simulink model "batteryGridPV_v17"  (R2014a)
settings: Solver=ode23tb  StartTime=0.0  StopTime=86400  MaxStep=0.2  RelTol=1e-5
PreLoadFcn:
  | % -- Recommended Settings --
  | %
  | %  Simulink:
  | %      Solver: Ode23tb
  | %      Relative tolerance = 1e-4
  | %      Max step size = 0.2
  | %
  | %  Powergui:
  |          Ts = 0; % (continuous electrical model)
  | %
  | %
  | % ----------------------------------
InitFcn:
  | Ncell = 80;
  | PVCellIsc = 7;
  | PVCellVoc = 0.64;
  | PVCellRs = 0.001;
  | tau = 1e-4;
  | 
  | initializeBattery();
StopFcn:
  | %plotSimResults();
values from neighbouring files (symbols this model uses):
  ambientTemp = 20    [initialConditions.m]    (also in initializeBattery.m)
  currentSat = 0.5    [controlParams.m]    (also in initializeBattery.m)
  desiredBusVoltage = 30    [controlParams.m]    (also in initializeBattery.m = 24.45)
  finalVoltage = 30    [controlParams.m]    (also in initializeBattery.m = 26)
  maxChargeRate = 5    [controlParams.m]    (also in initializeBattery.m)
  maxDischargeRate = -5    [controlParams.m]    (also in initializeBattery.m)
  T_init = ambientTemp + 273.15    (= 293.15)    [initialConditions.m]    (also in initializeBattery.m)
undefined symbols (not defined in the file or in its folder): Ion, Lithium
undefined symbols (not defined in the file): C1_LUT, C2_LUT, Capacity_LUT, cell_Cp_heat, cell_mass, Em_LUT, Qe_init, R0_LUT, R1_LUT, R2_LUT, SOC_LUT, Temperature_LUT
libraries: powerlib x42, fl_lib x18, nesl_utility x6, LiBatteryElements_lib x6, simulink x3, simulink_extras x3, electricdrivelib x1
(part 2 of 2)

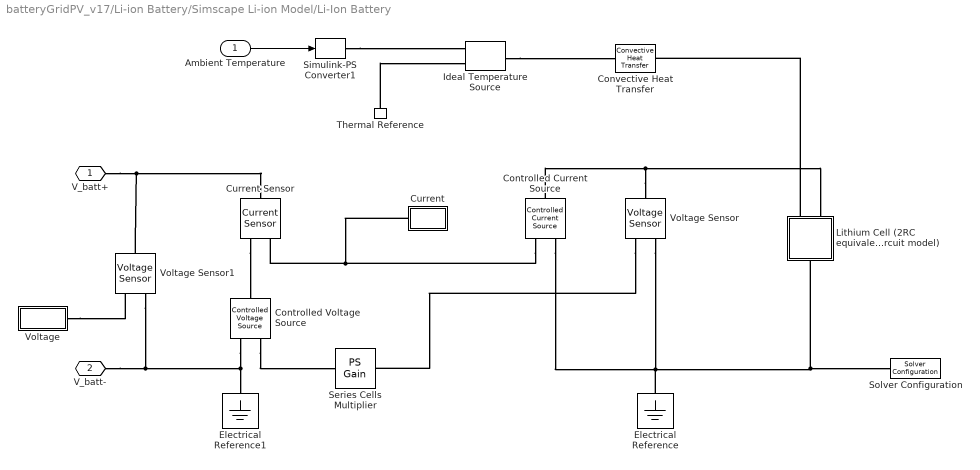
== system batteryGridPV_v17/Li-ion Battery/Simscape Li-ion Model/Li-Ion Battery ==
  Ambient Temperature : Inport
  Controlled Current Source : fl_lib/Electrical/Electrical Sources/Controlled Current Source
  Controlled Voltage Source : fl_lib/Electrical/Electrical Sources/Controlled Voltage Source
  Convective Heat Transfer : fl_lib/Thermal/Thermal Elements/Convective Heat Transfer  area=cell_area m^2  heat_tr_coeff=h_conv W/(m^2 * K)  Q_specify=off  Q_priority=High  Q=0 J/s  T_specify=off  T_priority=High  T=0 K
  Current : Subsystem
  Current Sensor : fl_lib/Electrical/Electrical Sensors/Current Sensor
  Electrical Reference : fl_lib/Electrical/Electrical Elements/Electrical Reference
  Electrical Reference1 : fl_lib/Electrical/Electrical Elements/Electrical Reference
  Ideal Temperature Source : fl_lib/Thermal/Thermal Sources/Ideal Temperature Source
  Lithium Cell (2RC equivalent circuit model) : Subsystem  mask(Lithium battery (two RC-branch equivalent circuit)){Qe_init=Qe_init, T_init=T_init, Capacity_LUT=Capacity_LUT, Em_LUT=Em_LUT, R0_LUT=R0_LUT, R1_LUT=R1_LUT, C1_LUT=C1_LUT, R2_LUT=R2_LUT, C2_LUT=C2_LUT, cell_mass=cell_mass, cell_Cp_heat=cell_Cp_heat, SOC_LUT=SOC_LUT, Temperature_LUT=Temperature_LUT}
      mask prompts: Qe_init "Initial charge deficit (A*hr)"; T_init "Initial cell temperature (K)"; Capacity_LUT "Capacity (A*hr, 1xN table)"; Em_LUT "Em open-circuit voltage (volts, MxN table)"; R0_LUT "R0 terminal resistance (ohms, MxN table)"; R1_LUT "R1 resistance (ohms, MxN table)"; C1_LUT "C1 capacitance (farads, MxN table)"; R2_LUT "R2 resistance (ohms, MxN table)"; C2_LUT "C2 capacitance (farads, MxN table)"; cell_mass "Cell mass (kg)"; cell_Cp_heat "Cell specific heat (J/kg/K)"; SOC_LUT "SOC table breakpoints (Mx1 array)"; Temperature_LUT "Temperature table breakpoints(K, 1xN array)"
      mask Display:
      | image(imread('battery.jpg'))
      | color('red')
      | port_label('LConn',1,'H')
      | port_label('LConn',2,'+')
      | port_label('RConn',1,'-')
  Series Cells Multiplier : fl_lib/Physical Signals/Functions/PS Gain  gain=7
  Simulink-PS Converter1 : nesl_utility/Simulink-PS Converter  PhysicalDomain=network_engine_domain  SubClassName=ps_input  LeftPortType=input  RightPortType=output  PseudoPeriodic=off  Frequencies=[]  NoiseDistribution=none  NoiseParameters=[]  Unit=C  AffineConversion=on  InputFiltering=off  SimscapeFilterOrder=1  InputFilterTimeConstant=.001  UdotUserProvided=1
  Solver Configuration : nesl_utility/Solver Configuration  PhysicalDomain=network_engine_domain  SubClassName=solver  LeftPortType=input  RightPortType=generic  Accelerate=off  Tones=[]  Harmonics=[]  SimulateNoise=off  Profile=off  UseLocalSampling=off  EnableSwitchedLinearOptims=on  FrequencyDomain=off  UseCCode=off  RelTol=0.001  AbsTol=1e-06  MinStep=1e-09  ToWorkspace=off  DoDC=on  ResidualTolerance=1e-9  UseLocalSolver=off  LocalSolverChoice=NE_BACKWARD_EULER_ADVANCER  LocalSolverSampleTime=1  DoFixedCost=off  MaxNonlinIter=3  MaxModeIter=2  LinearAlgebra=Sparse  DelaysMemoryBudget=1024  AutomaticFiltering=on  FilteringTimeConstant=0.001
  Thermal Reference : fl_lib/Thermal/Thermal Elements/Thermal Reference
  Voltage : Subsystem
  Voltage Sensor : fl_lib/Electrical/Electrical Sensors/Voltage Sensor
  Voltage Sensor1 : fl_lib/Electrical/Electrical Sensors/Voltage Sensor
  V_batt+ : PMIOPort  Port=1  Side=Left
  V_batt- : PMIOPort  Port=2  Side=Left
  wires:
  Ambient Temperature/1 -> Simulink-PS Converter1/1
  connections:
  V_batt+/RConn1 -- Voltage Sensor1/LConn1 -- Current Sensor/LConn1
  Controlled Voltage Source/RConn2 -- Voltage Sensor1/RConn2 -- V_batt-/RConn1 -- Electrical Reference1/LConn1
  Lithium Cell (2RC equivalent circuit model)/LConn1 -- Convective Heat Transfer/RConn1
  Thermal Reference/LConn1 -- Ideal Temperature Source/RConn2
  Simulink-PS Converter1/RConn1 -- Ideal Temperature Source/RConn1
  Ideal Temperature Source/LConn1 -- Convective Heat Transfer/LConn1
  Electrical Reference/LConn1 -- Lithium Cell (2RC equivalent circuit model)/RConn1 -- Solver Configuration/RConn1 -- Controlled Current Source/RConn2 -- Voltage Sensor/RConn2
  Controlled Current Source/RConn1 -- Current Sensor/RConn1 -- Current/RConn1
  Controlled Voltage Source/RConn1 -- Series Cells Multiplier/RConn1
  Voltage Sensor/LConn1 -- Lithium Cell (2RC equivalent circuit model)/LConn2 -- Controlled Current Source/LConn1
  Current Sensor/RConn2 -- Controlled Voltage Source/LConn1
  Voltage Sensor/RConn1 -- Series Cells Multiplier/LConn1
  Voltage/RConn1 -- Voltage Sensor1/RConn1

== system batteryGridPV_v17/PV//Battery Power Converters/Buck Converter/scaling ==
  note: Shifting from ]0 to 1[ to a ]-1 to 1[ scale
  D : Inport
  Bias : Bias  Bias=-0.5
  Gain : Gain  Gain=2
  Saturation : Saturate  UpperLimit=1  LowerLimit=-1
  m : Outport
  wires:
  Bias/1 -> Gain/1
  D/1 -> Bias/1
  Gain/1 -> Saturation/1
  Saturation/1 -> m/1

== system batteryGridPV_v17/Battery//PV Management and Control/Battery Charge//Discharge Controllers/Battery Charge Controller/scaling ==
  note: Shifting from ]0 to 1[ to a ]-1 to 1[ scale
  D : Inport
  Bias : Bias  Bias=-0.5
  Gain : Gain  Gain=2
  Saturation : Saturate  UpperLimit=1  LowerLimit=-1
  m : Outport
  wires:
  Saturation/1 -> m/1
  Gain/1 -> Saturation/1
  D/1 -> Bias/1
  Bias/1 -> Gain/1

== system batteryGridPV_v17/Battery//PV Management and Control/Battery Charge//Discharge Controllers/Battery Discharge Controller/scaling ==
  note: Shifting from ]0 to 1[ to a ]-1 to 1[ scale
  D : Inport
  Bias : Bias  Bias=-0.5
  Gain : Gain  Gain=-2
  Saturation : Saturate  UpperLimit=1  LowerLimit=-1
  m : Outport
  wires:
  Saturation/1 -> m/1
  Gain/1 -> Saturation/1
  D/1 -> Bias/1
  Bias/1 -> Gain/1

== system batteryGridPV_v17/Li-ion Battery/Simscape Li-ion Model/Li-Ion Battery/Current ==
  PS-Simulink Converter1 : nesl_utility/PS-Simulink Converter  PhysicalDomain=network_engine_domain  SubClassName=ps_output  LeftPortType=input  RightPortType=output  PseudoPeriodic=off  Frequencies=[]  Unit=A  AffineConversion=off
  PS : PMIOPort  Port=1  Side=Right
  tag scope: I_load=global
  wires:
  PS-Simulink Converter1/1 -> [I_load]
  connections:
  PS-Simulink Converter1/LConn1 -- PS/RConn1

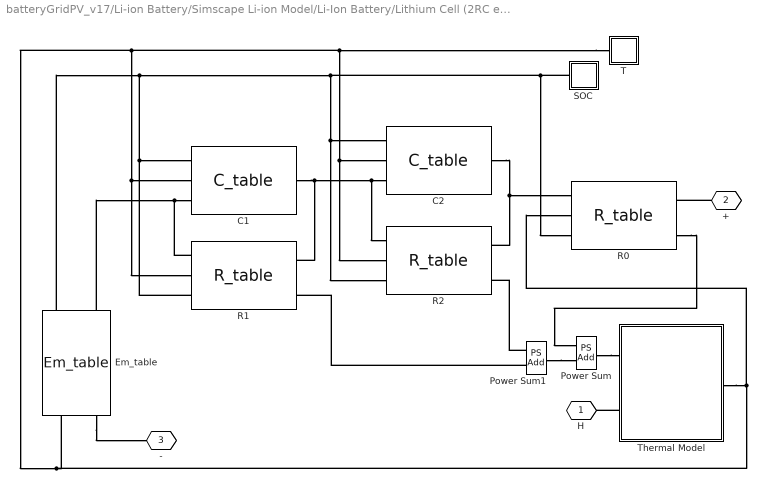
== system batteryGridPV_v17/Li-ion Battery/Simscape Li-ion Model/Li-Ion Battery/Lithium Cell (2RC equivalent circuit model) ==
  " SOC " : Subsystem
  C1 : LiBatteryElements_lib/C_table  C_Table=C1_LUT F  SOC_Table=SOC_LUT  Temp_Table=Temperature_LUT K  v0=0 V
  C2 : LiBatteryElements_lib/C_table  C_Table=C2_LUT F  SOC_Table=SOC_LUT  Temp_Table=Temperature_LUT K  v0=0 V
  Em_table : LiBatteryElements_lib/Em_table  C_Table=Capacity_LUT hr*A  Em_Table=Em_LUT V  SOC_Table=SOC_LUT  Temp_Table=Temperature_LUT K  Qinit=Qe_init hr*A
  Power Sum : fl_lib/Physical Signals/Functions/PS Add
  Power Sum1 : fl_lib/Physical Signals/Functions/PS Add
  R0 : LiBatteryElements_lib/R_table  R_Table=R0_LUT Ohm  SOC_Table=SOC_LUT  Temp_Table=Temperature_LUT K
  R1 : LiBatteryElements_lib/R_table  R_Table=R1_LUT Ohm  SOC_Table=SOC_LUT  Temp_Table=Temperature_LUT K
  R2 : LiBatteryElements_lib/R_table  R_Table=R2_LUT Ohm  SOC_Table=SOC_LUT  Temp_Table=Temperature_LUT K
  T : Subsystem
  Thermal Model : Subsystem
  H : PMIOPort  Tag=PMCPort  Port=1  Side=Left
  + : PMIOPort  Tag=PMCPort  Port=2  Side=Left
  - : PMIOPort  Tag=PMCPort  Port=3  Side=Right
  connections:
  Thermal Model/LConn2 -- H/RConn1
  Em_table/RConn1 -- -/RConn1
  +/RConn1 -- R0/RConn1
  Em_table/LConn1 -- R1/LConn1 -- C1/LConn1
  T/LConn1 -- Thermal Model/RConn1 -- R0/LConn2 -- Em_table/RConn2 -- C1/LConn2 -- R1/LConn2 -- C2/LConn2 -- R2/LConn2
  Power Sum/RConn1 -- Thermal Model/LConn1
  R1/RConn1 -- R2/LConn1 -- C2/LConn1 -- C1/RConn1
  R0/RConn2 -- Power Sum/LConn1
  Power Sum1/RConn1 -- Power Sum/LConn2
  C2/RConn1 -- R0/LConn1 -- R2/RConn1
  Power Sum1/LConn1 -- R2/RConn2
  R1/LConn3 -- C1/LConn3 -- " SOC "/LConn1 -- R0/LConn3 -- C2/LConn3 -- R2/LConn3 -- Em_table/LConn3
  Power Sum1/LConn2 -- R1/RConn2

== system batteryGridPV_v17/Li-ion Battery/Simscape Li-ion Model/Li-Ion Battery/Voltage ==
  PS-Simulink Converter : nesl_utility/PS-Simulink Converter  PhysicalDomain=network_engine_domain  SubClassName=ps_output  LeftPortType=input  RightPortType=output  PseudoPeriodic=off  Frequencies=[]  Unit=V  AffineConversion=off
  PS : PMIOPort  Port=1  Side=Right
  tag scope: V_load=global
  wires:
  PS-Simulink Converter/1 -> [V_load]
  connections:
  PS-Simulink Converter/LConn1 -- PS/RConn1

== system batteryGridPV_v17/Li-ion Battery/Simscape Li-ion Model/Li-Ion Battery/Lithium Cell (2RC equivalent circuit model)/ SOC  ==
  PS-Simulink Converter1 : nesl_utility/PS-Simulink Converter  PhysicalDomain=network_engine_domain  SubClassName=ps_output  LeftPortType=input  RightPortType=output  PseudoPeriodic=off  Frequencies=[]  Unit=1  AffineConversion=off
  PS : PMIOPort  Port=1  Side=Left
  tag scope: SOC=global
  wires:
  PS-Simulink Converter1/1 -> [SOC]
  connections:
  PS/RConn1 -- PS-Simulink Converter1/LConn1

== system batteryGridPV_v17/Li-ion Battery/Simscape Li-ion Model/Li-Ion Battery/Lithium Cell (2RC equivalent circuit model)/T ==
  PS-Simulink Converter1 : nesl_utility/PS-Simulink Converter  PhysicalDomain=network_engine_domain  SubClassName=ps_output  LeftPortType=input  RightPortType=output  PseudoPeriodic=off  Frequencies=[]  Unit=C  AffineConversion=on
  PS : PMIOPort  Port=1  Side=Left
  tag scope: T=global
  wires:
  PS-Simulink Converter1/1 -> [T]
  connections:
  PS/RConn1 -- PS-Simulink Converter1/LConn1

== system batteryGridPV_v17/Li-ion Battery/Simscape Li-ion Model/Li-Ion Battery/Lithium Cell (2RC equivalent circuit model)/Thermal Model ==
  Battery thermal mass : fl_lib/Thermal/Thermal Elements/Thermal Mass  mass=cell_mass kg  sp_heat=cell_Cp_heat J/kg/K  Q_specify=off  Q_priority=High  Q=0 J/s  T_specify=on  T_priority=High  T=T_init K
  Ideal Temperature Sensor : fl_lib/Thermal/Thermal Sensors/Ideal Temperature Sensor
  Ideal Heat Flow Source : fl_lib/Thermal/Thermal Sources/Ideal Heat Flow Source
  Thermal Reference1 : fl_lib/Thermal/Thermal Elements/Thermal Reference
  Thermal Reference2 : fl_lib/Thermal/Thermal Elements/Thermal Reference
  P_in : PMIOPort  Tag=PMCPort  Port=1  Side=Left
  H : PMIOPort  Tag=PMCPort  Port=2  Side=Left
  T : PMIOPort  Tag=PMCPort  Port=3  Side=Right
  connections:
  Thermal Reference2/LConn1 -- Ideal Temperature Sensor/RConn1
  Ideal Temperature Sensor/RConn2 -- T/RConn1
  Thermal Reference1/LConn1 -- Ideal Heat Flow Source/RConn2
  Ideal Temperature Sensor/LConn1 -- H/RConn1 -- Battery thermal mass/LConn1 -- Ideal Heat Flow Source/LConn1
  Ideal Heat Flow Source/RConn1 -- P_in/RConn1

== stateflow chart batteryGridPV_v17/Battery//PV Management and Control/Battery Mode Selection ==
  note: Simple switch logic for charge/discharge operation
      |   - Can be readily expanded through Stateflow
      |   - Incorporate information on grid/PV availability
      |   - Future work: optimization to determine ideal mode
  state dischargeMode
    during:
    batteryMode = 0;
    controlOnOff = 1;
    state constantVoltage
      during:
      controlSelect = 1;
      batteryDisengage = 0;
    state constantCurrent
      during:
      controlSelect = 0;
      batteryDisengage = 0;
    (default) -> dischargeMode.constantVoltage : {dischargeHysteresis = 1e-1;}
    dischargeMode.constantVoltage -> dischargeMode.constantCurrent : [measures.Bus.BattCurrent <= maxDischargeRate]
    dischargeMode.constantCurrent -> dischargeMode.constantVoltage : [measures.Bus.BattCurrent > maxDischargeRate + dischargeHysteresis || ...
        | measures.Bus.BusVoltage > desiredBusVoltage + dischargeHysteresis ]
  state chargeMode
    during:
    batteryMode = 1;
    controlOnOff = 1;
    state constantVoltage
      during:
      controlSelect = 0;
      batteryDisengage = 0;
    state constantCurrent
      during:
      controlSelect = 1;
      batteryDisengage = 0;
    state currentSaturate
      during:
      controlSelect = 0;
      batteryDisengage = 1;
    (default) -> chargeMode.constantCurrent : {chargeHysteresis = 0.1;}
    chargeMode.constantCurrent -> chargeMode.constantVoltage : [finalVoltage <= measures.Bus.BattVoltage]
    chargeMode.constantVoltage -> currentSaturate [order 2] : [measures.Bus.BattCurrent <= currentSat]
    chargeMode.constantVoltage -> chargeMode.constantCurrent [order 1] : [finalVoltage > measures.Bus.BattVoltage + chargeHysteresis ]
  state disableMode
    during:
    batteryMode = 1;
    controlOnOff = 0;
  (default) -> chargeMode : {batteryDisengage = 0;}
  chargeMode -> dischargeMode [order 1] : [(measures.PV.Power < measures.Load.Power || ...
      |  measures.Battery.Current < 0) && ...
      | after(5, sec)]
  dischargeMode -> chargeMode [order 1] : [measures.PV.Power > measures.Load.Power  && ...
      | after(5, sec)]
  chargeMode -> disableMode [order 2] : [switches.battery == 1 || ...
      | batteryDisengage == 1]
  dischargeMode -> disableMode [order 2] : [switches.pv ~= 1]
  disableMode -> dischargeMode : [(switches.battery == 0 && batteryDisengage == 0) || ...
      |  (switches.battery == 0 &&  measures.PV.Power < measures.Load.Power) || ...
      | switches.pv == 1]{batteryDisengage = 0;}
  data: controlOnOff output; switches input; batteryMode output; batteryDisengage local; chargeHysteresis local; dischargeHysteresis local; currentSat parameter; finalVoltage parameter; controlSelect output; maxDischargeRate parameter; desiredBusVoltage parameter; measures input Bus: Measurements
